simulink model "SerialMonitorScope"  (R2016b)
settings: Solver=FixedStepDiscrete  StartTime=0.0  StopTime=inf  FixedStep=Tsa  RelTol=1e-3  EnableMultiTasking=on
StartFcn:
  | s_2 = serial(Port1,'BaudRate',115200,'FlowControl','none','Parity','none','DataBits',8,'StopBits',1,'Timeout',2);
  | s_2.InputBufferSize=1024*5; s_2.OutputBufferSize=1024*5;
  | s_2.Terminator='CR';
  | 
  | fopen(s_2);
StopFcn:
  | fclose(s_2);
values from neighbouring files (symbols this model uses):
  TCommand = 1    [TempControlSysId.mat]
  Tsa = 1    [TempControlSysId.mat]
undefined symbols (not defined in the file or in its folder): serialMonitorRead, serialMonitorWrite
libraries: sldrtlib x1
settings Model: Creator=EliteBook 8470p  LastModifiedBy=rsjoshi1
settings DataIOCC: LimitDataPoints=on  SaveFormat=Array
settings OptimizationCC: LifeSpan=inf
settings DebuggingCC: SolverPrmCheckMsg=warning  SFUnexpectedBacktrackingDiag=warning  SFNoUnconditionalDefaultTransitionDiag=warning  SFExecutionAtInitializationDiag=none
settings HardwareCC: ProdBitPerPointer=32  ProdBitPerSizeT=32  ProdBitPerPtrDiffT=32  ProdLargestAtomicFloat=None  ProdIntDivRoundTo=Undefined  ProdEndianess=Unspecified  ProdWordSize=32  ProdHWDeviceType=32-bit Generic
settings ModelReferenceCC: PropagateSignalLabelsOutOfModel=off
settings GRTTargetCC: TargetLangStandard=C89/C90 (ANSI)  GeneratePreprocessorConditionals=Disable all
settings ConfigComp: CovMetricSettings=dw  CovHtmlReporting=on  CovSaveCumulativeToWorkspaceVar=on  CovSaveSingleToWorkspaceVar=on  CovExternalEMLEnable=off  CovSFcnEnable=off

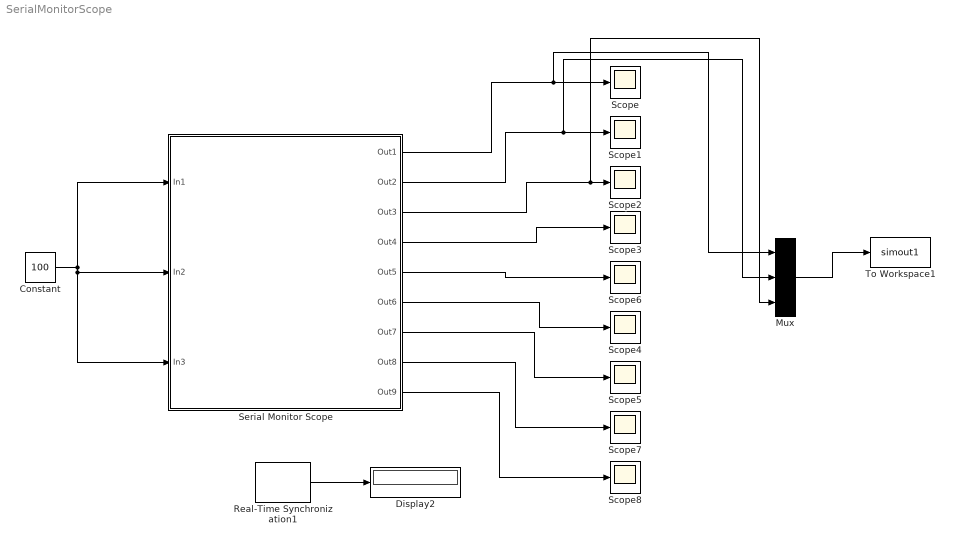
== system SerialMonitorScope ==
  Constant : Constant  Value=100  SampleTime=Tsa
  Display2 : Display
  Mux : Mux  Inputs=3
  Real-Time Synchronization1 : sldrtlib/Real-Time Synchronization  SampleTime=Tsa  MaxMissedTicks=5000  ShowMissedTicks=on  YieldWhenWaiting=off
  Scope{,1..8} (9 alike) : Scope
  Serial Monitor Scope : Subsystem  Description=Serial Monitor Scope
  To Workspace1 : ToWorkspace  VariableName=simout1  SaveFormat=Timeseries  SampleTime=-1
  wires:
  Real-Time Synchronization1/1 -> Display2/1
  Serial Monitor Scope/1(Out1) -> Mux/1, Scope/1
  Serial Monitor Scope/2(Out2) -> Mux/2, Scope1/1
  Serial Monitor Scope/3(Out3) -> Mux/3, Scope2/1
  Serial Monitor Scope/4(Out4) -> Scope3/1
  Serial Monitor Scope/5(Out5) -> Scope6/1
  Serial Monitor Scope/6(Out6) -> Scope4/1
  Serial Monitor Scope/7(Out7) -> Scope5/1
  Serial Monitor Scope/8(Out8) -> Scope7/1
  Serial Monitor Scope/9(Out9) -> Scope8/1
  Constant/1 -> Serial Monitor Scope/2(In2), Serial Monitor Scope/3(In3), Serial Monitor Scope/1(In1)
  Mux/1 -> To Workspace1/1

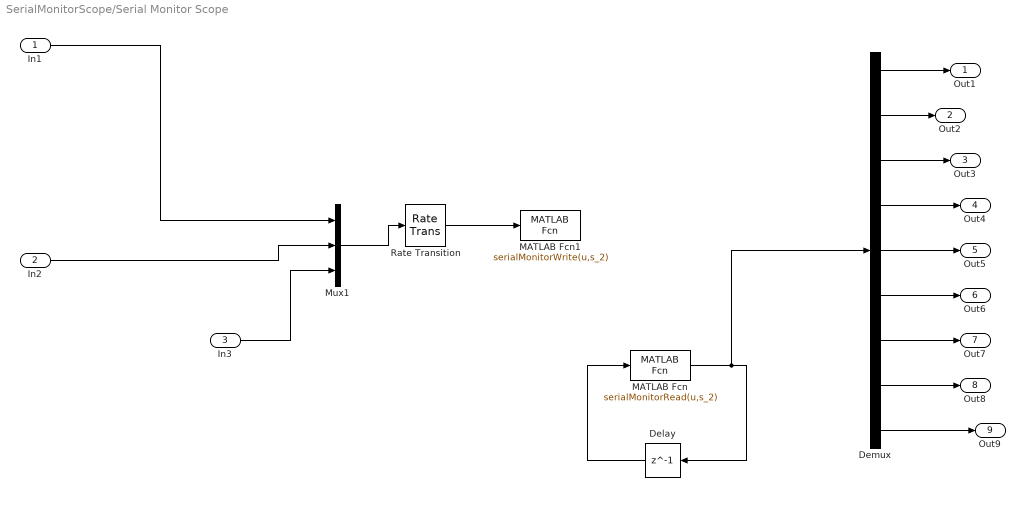
== system SerialMonitorScope/Serial Monitor Scope ==
  In1 : Inport
  In2 : Inport  Port=2
  In3 : Inport  Port=3
  Delay : Delay  DelayLength=1  InitialCondition=0  SampleTime=Tsa
  Demux : Demux  Outputs=9
  MATLAB Fcn : MATLABFcn  MATLABFcn=serialMonitorRead(u,s_2)  OutputDimensions=9
  MATLAB Fcn1 : MATLABFcn  MATLABFcn=serialMonitorWrite(u,s_2)  OutputDimensions=0
  Mux1 : Mux  Inputs=3
  Rate Transition : RateTransition  Deterministic=off  OutPortSampleTime=Tsa*TCommand
  Out1 : Outport
  Out2 : Outport  Port=2
  Out3 : Outport  Port=3
  Out4 : Outport  Port=4
  Out5 : Outport  Port=5
  Out6 : Outport  Port=6
  Out7 : Outport  Port=7
  Out8 : Outport  Port=8
  Out9 : Outport  Port=9
  wires:
  Mux1/1 -> Rate Transition/1
  Rate Transition/1 -> MATLAB Fcn1/1
  In1/1 -> Mux1/1
  In3/1 -> Mux1/3
  In2/1 -> Mux1/2
  Delay/1 -> MATLAB Fcn/1
  MATLAB Fcn/1 -> Demux/1, Delay/1
  Demux/1 -> Out1/1
  Demux/9 -> Out9/1
  Demux/8 -> Out8/1
  Demux/7 -> Out7/1
  Demux/6 -> Out6/1
  Demux/5 -> Out5/1
  Demux/4 -> Out4/1
  Demux/3 -> Out3/1
  Demux/2 -> Out2/1
